simulink model "simulink_model"  (R2013b)
settings: Solver=ode45  StartTime=0.0  StopTime=30  RelTol=1e-3
settings Model: Creator=petter  LastModifiedBy=petter

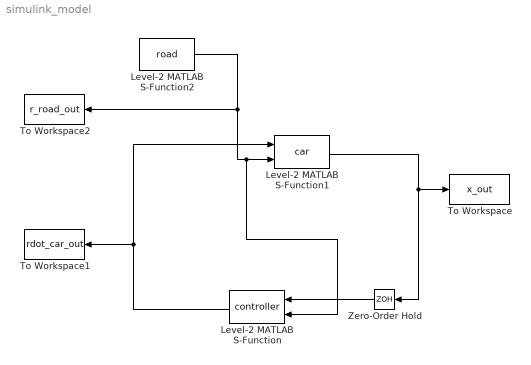
== system simulink_model ==
  Level-2 MATLAB S-Function : M-S-Function  FunctionName=controller  Parameters=1
  Level-2 MATLAB S-Function1 : M-S-Function  FunctionName=car
  Level-2 MATLAB S-Function2 : M-S-Function  FunctionName=road
  To Workspace : ToWorkspace  VariableName=x_out  SampleTime=-1  SaveFormat=Structure With Time
  To Workspace1 : ToWorkspace  VariableName=rdot_car_out  SampleTime=-1  SaveFormat=Structure With Time
  To Workspace2 : ToWorkspace  VariableName=r_road_out  SampleTime=-1  SaveFormat=Structure With Time
  Zero-Order Hold : ZeroOrderHold  SampleTime=0.1
  wires:
  Level-2 MATLAB S-Function1/1 -> Zero-Order Hold/1, To Workspace/1
  Level-2 MATLAB S-Function/1 -> Level-2 MATLAB S-Function1/1, To Workspace1/1
  Level-2 MATLAB S-Function2/1 -> To Workspace2/1, Level-2 MATLAB S-Function/2, Level-2 MATLAB S-Function1/2
  Zero-Order Hold/1 -> Level-2 MATLAB S-Function/1
